simulink model "ssp_ad_scan"  (Simulink 6.5)
settings: Solver=VariableStepDiscrete  SolverMode=SingleTasking  StartTime=0.0  StopTime=10  RelTol=1e-3
undefined symbols (not defined in the file or in its folder): gcbh, xlBlockLoadCallback, xlGetSimulinkPeriod
libraries: xbsIndex_r4 x111, nort_sysgenlib x19
(part 2 of 2)

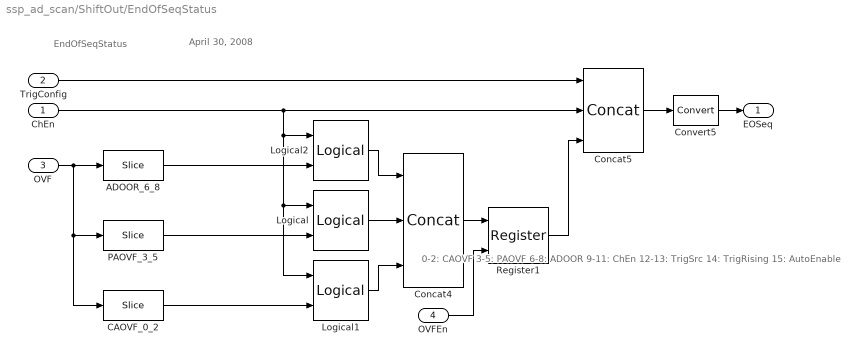
== system ssp_ad_scan/ShiftOut/EndOfSeqStatus ==
  note: EndOfSeqStatus
  note: April 30, 2008
  note: 0-2: CAOVF
      | 3-5: PAOVF
      | 6-8: ADOOR
      | 9-11: ChEn
      | 12-13: TrigSrc
      | 14: TrigRising
      | 15: AutoEnable
  ChEn : Inport
  TrigConfig : Inport  Port=2
  OVF : Inport  Port=3
  OVFEn : Inport  Port=4
  ADOOR_6_8 : xbsIndex_r4/Slice  nbits=3  boolean_output=off  mode=Lower Bit Location + Width  bit1=0  base1=MSB of Input  bit0=6  base0=LSB of Input  dbl_ovrd=off  block_type=slice
      settings: infoedit="Extracts a given range of bits from each input sample and presents it at the output.  The output type is ordinarily unsigned with binary point at zero, but can be Boolean when the slice is one bit wide.<P><P>Hardware notes: In hardware this block costs nothing."  block_version=9.2.01
  CAOVF_0_2 : xbsIndex_r4/Slice  nbits=3  boolean_output=off  mode=Lower Bit Location + Width  bit1=0  base1=MSB of Input  bit0=0  base0=LSB of Input  dbl_ovrd=off  block_type=slice
      settings: infoedit="Extracts a given range of bits from each input sample and presents it at the output.  The output type is ordinarily unsigned with binary point at zero, but can be Boolean when the slice is one bit wide.<P><P>Hardware notes: In hardware this block costs nothing."  block_version=9.2.01
  Concat4 : xbsIndex_r4/Concat  num_inputs=3  dbl_ovrd=off  block_type=concat
      settings: block_version=9.2.01
  Concat5 : xbsIndex_r4/Concat  num_inputs=3  dbl_ovrd=off  block_type=concat
      settings: block_version=9.2.01
  Convert5 : xbsIndex_r4/Convert  arith_type=Unsigned  n_bits=32  bin_pt=0  quantization=Truncate  overflow=Wrap  latency=0  dbl_ovrd=off  pipeline=off  block_type=convert
      settings: block_version=9.2.01
  Logical : xbsIndex_r4/Logical  logical_function=AND  inputs=2  en=off  latency=0  precision=Full  arith_type=Unsigned  n_bits=16  bin_pt=0  align_bp=on  dbl_ovrd=off  block_type=logical
      settings: block_version=9.2.01
  Logical1 : xbsIndex_r4/Logical  logical_function=AND  inputs=2  en=off  latency=0  precision=Full  arith_type=Unsigned  n_bits=16  bin_pt=0  align_bp=on  dbl_ovrd=off  block_type=logical
      settings: block_version=9.2.01
  Logical2 : xbsIndex_r4/Logical  logical_function=AND  inputs=2  en=off  latency=0  precision=Full  arith_type=Unsigned  n_bits=16  bin_pt=0  align_bp=on  dbl_ovrd=off  block_type=logical
      settings: block_version=9.2.01
  PAOVF_3_5 : xbsIndex_r4/Slice  nbits=3  boolean_output=off  mode=Lower Bit Location + Width  bit1=0  base1=MSB of Input  bit0=3  base0=LSB of Input  dbl_ovrd=off  block_type=slice
      settings: infoedit="Extracts a given range of bits from each input sample and presents it at the output.  The output type is ordinarily unsigned with binary point at zero, but can be Boolean when the slice is one bit wide.<P><P>Hardware notes: In hardware this block costs nothing."  block_version=9.2.01
  Register1 : xbsIndex_r4/Register  init=0  rst=off  en=on  dbl_ovrd=off  block_type=register
      settings: block_version=9.2.01
  EOSeq : Outport
  wires:
  Concat4/1 -> Register1/1
  Register1/1 -> Concat5/3
  Concat5/1 -> Convert5/1
  ChEn/1 -> Logical/1, Logical1/1, Logical2/1, Concat5/2
  TrigConfig/1 -> Concat5/1
  Convert5/1 -> EOSeq/1
  OVFEn/1 -> Register1/2
  Logical/1 -> Concat4/2
  OVF/1 -> ADOOR_6_8/1, CAOVF_0_2/1, PAOVF_3_5/1
  Logical1/1 -> Concat4/3
  ADOOR_6_8/1 -> Logical2/2
  PAOVF_3_5/1 -> Logical/2
  Logical2/1 -> Concat4/1
  CAOVF_0_2/1 -> Logical1/2

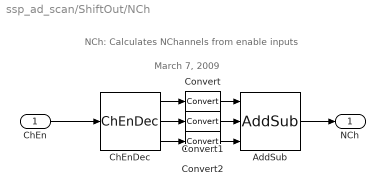
== system ssp_ad_scan/ShiftOut/NCh ==
  note: NCh: Calculates NChannels from enable inputs
  note: March 7, 2009
  ChEn : Inport
  AddSub : xbsIndex_r4/AddSub  mode=Addition  use_carryin=on  use_carryout=off  en=off  latency=0  precision=User Defined  arith_type=Unsigned  n_bits=16  bin_pt=0  quantization=Truncate  overflow=Wrap  dbl_ovrd=off  use_behavioral_HDL=off  pipelined=off  use_rpm=on  block_type=addsub
      settings: block_version=9.2.01
  ChEnDec : nort_sysgenlib/ChEnDec  SystemSampleTime=-1
  Convert : xbsIndex_r4/Convert  arith_type=Unsigned  n_bits=1  bin_pt=0  quantization=Truncate  overflow=Wrap  latency=0  dbl_ovrd=off  pipeline=off  block_type=convert
      settings: block_version=9.2.01
  Convert1 : xbsIndex_r4/Convert  arith_type=Unsigned  n_bits=1  bin_pt=0  quantization=Truncate  overflow=Wrap  latency=0  dbl_ovrd=off  pipeline=off  block_type=convert
      settings: block_version=9.2.01
  Convert2 : xbsIndex_r4/Convert  arith_type=Unsigned  n_bits=1  bin_pt=0  quantization=Truncate  overflow=Wrap  latency=0  dbl_ovrd=off  pipeline=off  block_type=convert
      settings: block_version=9.2.01
  NCh : Outport
  wires:
  AddSub/1 -> NCh/1
  ChEn/1 -> ChEnDec/1
  ChEnDec/1 -> Convert/1
  ChEnDec/2 -> Convert1/1
  ChEnDec/3 -> Convert2/1
  Convert/1 -> AddSub/1
  Convert1/1 -> AddSub/2
  Convert2/1 -> AddSub/3

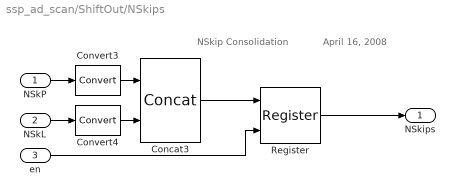
== system ssp_ad_scan/ShiftOut/NSkips ==
  note: NSkip Consolidation
  note: April 16, 2008
  NSkP : Inport
  NSkL : Inport  Port=2
  en : Inport  Port=3
  Concat3 : xbsIndex_r4/Concat  num_inputs=2  dbl_ovrd=off  block_type=concat
      settings: block_version=9.2.01
  Convert3 : xbsIndex_r4/Convert  arith_type=Unsigned  n_bits=16  bin_pt=0  quantization=Truncate  overflow=Wrap  latency=0  dbl_ovrd=off  pipeline=off  block_type=convert
      settings: block_version=9.2.01
  Convert4 : xbsIndex_r4/Convert  arith_type=Unsigned  n_bits=16  bin_pt=0  quantization=Truncate  overflow=Wrap  latency=0  dbl_ovrd=off  pipeline=off  block_type=convert
      settings: block_version=9.2.01
  Register : xbsIndex_r4/Register  init=0  rst=off  en=on  dbl_ovrd=off  block_type=register
      settings: block_version=9.2.01
  NSkips : Outport
  wires:
  Convert3/1 -> Concat3/1
  Convert4/1 -> Concat3/2
  NSkP/1 -> Convert3/1
  NSkL/1 -> Convert4/1
  Concat3/1 -> Register/1
  Register/1 -> NSkips/1
  en/1 -> Register/2
